simulink model "L1ZR5_Regelstrecke_inputgain_Modell_FRNEU"  (Simulink 7.8)
settings: Solver=ode45  StartTime=0.0  StopTime=10  FixedStep=6e-4
values from neighbouring files (symbols this model uses):
  Am = [0 1; -1/T^2 -2*xi/T]    [L1ZR5_Regelstrecke1_inputgain_Modell.m]    (also in Timedelaymargin.m = [0 1; -0.6400   -1.9200])
  b = [0;1]    [L1ZR5_Regelstrecke1_inputgain_Modell.m]    (also in Timedelaymargin.m)
  c = [1 0]    [L1ZR5_Regelstrecke1_inputgain_Modell.m]    (also in Timedelaymargin.m)
  epsilon = 1.3    [L1ZR5_Regelstrecke1_inputgain_Modell.m]
  epsilon_omega = 0.1    [L1ZR5_Regelstrecke1_inputgain_Modell.m]
  epsilon_sigma = 0.1    [L1ZR5_Regelstrecke1_inputgain_Modell.m]
  epsilon_theta = 0.1    [L1ZR5_Regelstrecke1_inputgain_Modell.m]
  Gamma = 100000000    [L1ZR5_Regelstrecke1_inputgain_Modell.m]
  ICy = 0    [L1ZR5_Regelstrecke1_inputgain_Modell.m]
  k = 1750    [L1ZR5_Regelstrecke1_inputgain_Modell.m]
  kg = -1/(c/Am*b)    [L1ZR5_Regelstrecke1_inputgain_Modell.m]
  KmY = 2.4    [L1ZR5_Regelstrecke1_inputgain_Modell.m]
  Kq = [(theta1_max+theta1_min)/2 (theta2_max+theta2_min)/2]    [L1ZR5_Regelstrecke1_inputgain_Modell.m]
  kvy = 0    [L1ZR5_Regelstrecke1_inputgain_Modell.m]
  m = 19    [L1ZR5_Regelstrecke1_inputgain_Modell.m]
  M = tf(ss(Am,bm,cm,0))    [L1ZR5_Regelstrecke1_inputgain_Modell.m]
  omega_max = omega0_max*1.2    (= 0.394105263158)    [L1ZR5_Regelstrecke1_inputgain_Modell.m]
  omega_min = omega0_min/1.2    (= 0.0311111111111)    [L1ZR5_Regelstrecke1_inputgain_Modell.m]
  omega_Pmax = (omega_max-omega_min)/2    (= 0.181497076023)    [L1ZR5_Regelstrecke1_inputgain_Modell.m]
  omega_Pr_Center = omega_Pmax + omega_min    (= 0.212608187135)    [L1ZR5_Regelstrecke1_inputgain_Modell.m]
  Pb = P*b    [L1ZR5_Regelstrecke1_inputgain_Modell.m]
  pD = p(2)-1.92    [L1ZR5_Regelstrecke1_inputgain_Modell.m]
  pI = p(4)    [L1ZR5_Regelstrecke1_inputgain_Modell.m]
  pK = p(3)-0.64    [L1ZR5_Regelstrecke1_inputgain_Modell.m]
  Ref_Amplitude = 0.3/Ref_Frequenz^2    (= 0.000303963550927)    [L1ZR5_Regelstrecke1_inputgain_Modell.m]
  Ref_Frequenz = 2*pi*5    (= 31.4159265359)    [L1ZR5_Regelstrecke1_inputgain_Modell.m]
  sigma_Pmax = Delta    (= 1000)    [L1ZR5_Regelstrecke1_inputgain_Modell.m]
  theta_Pmax = 2.56    [L1ZR5_Regelstrecke1_inputgain_Modell.m]
undefined symbols (not defined in the file or in its folder): d1, d2, delta, FpxLookUp1, FpxLookUp2, FpyLookUp1, FpyLookUp2, ICphi, ICvphi, ICvx, ICvy, ICx, J, KmX, kvphi, kvx, KX1, KX2, KY1, KY2, Ox1, Ox2, Oy1, Oy2, phx, phy, sigma, Tk, Vx1, Vx2, Vy1, Vy2, xLookUp1, xLookUp2, yLookUp1, yLookUp2
libraries: vrlib x6, simulink x3
settings Model: Creator=Markus  LastModifiedBy=Markus
settings SolverCC: ZeroCrossControl=EnableAll

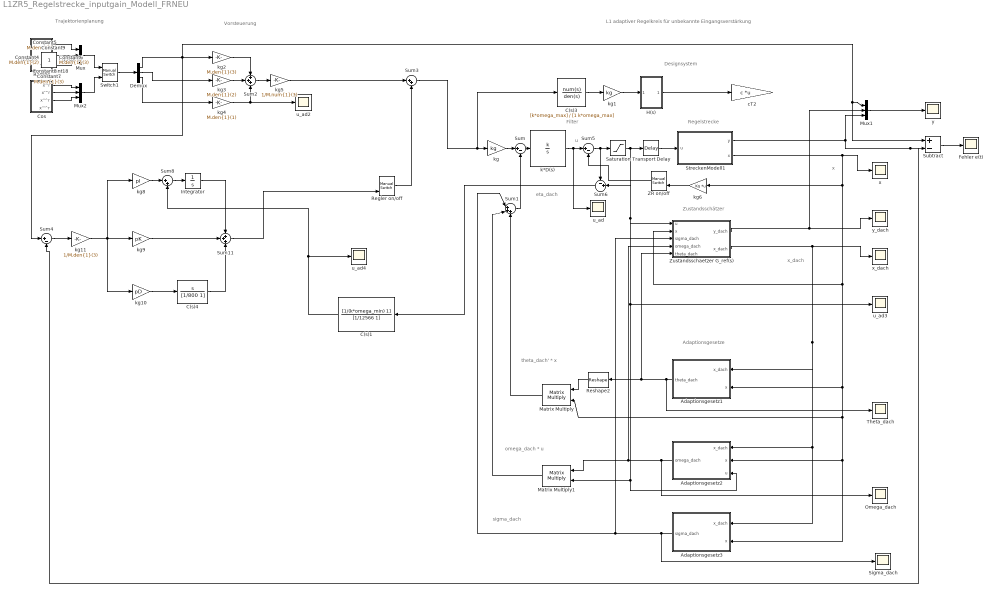
== system L1ZR5_Regelstrecke_inputgain_Modell_FRNEU ==
  note: Regelstrecke
  note: Zustandsschätzer
  note: Adaptionsgesetze
  note: L1 adaptiver Regelkreis für unbekannte Eingangsverstärkung
  note: x_dach
  note: x
  note: Filter
  note: u
  note: Designsystem
  note: theta_dach' * x
  note: omega_dach * u
  note: sigma_dach
  note: eta_dach
  note: Vorsteuerung
  note: Trajektorienplanung
  Adaptionsgesetz1 : Subsystem
  Adaptionsgesetz2 : Subsystem
  Adaptionsgesetz3 : Subsystem
  C(s)1 : TransferFcn  Numerator=[1/(k*omega_min) 1]  Denominator=[1/12566 1]
  C(s)3 : TransferFcn  Numerator=[k*omega_max]  Denominator=[1 k*omega_max]
  C(s)4 : TransferFcn  Numerator=[1 0]  Denominator=[1/800 1]
  Cos : Subsystem
  Demux : Demux  Outputs=3
  Fehler e(t) : Scope
      settings: TimeRange=4  YMin=-2.75e-005  YMax=2e-005  SaveName=simoutE
  H(s) : Subsystem
  Integrator : Integrator
  Matrix Multiply : Product  Multiplication=Matrix(*)
  Matrix Multiply1 : Product  Multiplication=Matrix(*)
  Mux : Mux  Inputs=3
  Mux1 : Mux  Inputs=3
  Mux2 : Mux  Inputs=3
  Omega_dach : Scope
      settings: TimeRange=0.01659605551497442  YMin=0.229945  YMax=0.254149  SaveName=simoutO
  Rampe : Subsystem
  Regler on/off : simulink/Signal Routing/Manual Switch  sw=0  action=0  varsize=off
  Reshape2 : Reshape  OutputDimensionality=Row vector (2-D)
  Saturation : Saturate  UpperLimit=20  LowerLimit=-20
  Sigma_dach : Scope
      settings: TimeRange=0.01659605551497442  YMin=0.18  YMax=0.25  SaveName=simoutS
  StreckenModell1 : Subsystem
  Subtract : Sum  Inputs=+-
  Sum : Sum  Inputs=|+-
  Sum1 : Sum  Inputs=|+++
  Sum11 : Sum  Inputs=+++
  Sum2 : Sum  Inputs=+++
  Sum3 : Sum  Inputs=|++
  Sum4 : Sum  Inputs=|+-
  Sum5 : Sum  Inputs=|+-
  Sum6 : Sum  Inputs=-+|
  Sum8 : Sum  Inputs=|++
  Switch1 : simulink/Signal Routing/Manual Switch  sw=1  action=0  varsize=off
  Theta_dach : Scope
      settings: TimeRange=0.01659605551497442  YMin=-0.05  YMax=0.275  SaveName=simoutT
  Transport Delay : TransportDelay  DelayTime=0.002
  ZR on/off : simulink/Signal Routing/Manual Switch  sw=1  action=0  varsize=off
  Zustandsschaetzer G_ref(s) : Subsystem
  cT2 : Gain  Gain=c  Multiplication=Matrix(K*u)
  k*D(s) : TransferFcn  Numerator=k  Denominator="[1  0]"
  kg : Gain  Gain=kg
  kg1 : Gain  Gain=kg
  kg10 : Gain  Gain=pD
  kg11 : Gain  Gain=1/M.den{1}(3)
  kg2 : Gain  Gain=M.den{1}(3)
  kg3 : Gain  Gain=M.den{1}(2)
  kg4 : Gain  Gain=M.den{1}(1)
  kg5 : Gain  Gain=1/M.num{1}(3)
  kg6 : Gain  Gain=Kq  Multiplication=Matrix(K*u)
  kg8 : Gain  Gain=pI
  kg9 : Gain  Gain=pK
  u_ad{,2..4} (4 alike) : Scope
      u_ad settings: TimeRange=4  YMin=-30  YMax=35  SaveName=simoutU
      u_ad2 settings: TimeRange=8  YMin=0.04404  YMax=0.04427  SaveName=simoutU2
      u_ad3 settings: TimeRange=4  YMin=-15  YMax=20  SaveName=simoutU3
      u_ad4 settings: TimeRange=20  YMin=-170  YMax=50  SaveName=simoutV2
  x : Scope
      settings: YMin=-0.0625  YMax=-0.005  SaveName=ScopeData3
  x_dach : Scope
      settings: YMin=-0.5  YMax=0.5  SaveName=ScopeData4
  y : Scope
      settings: TimeRange=4  YMin=-0.003  YMax=0.0015  SaveName=simout
  y_dach : Scope
      settings: YMin=0  YMax=35
  Constant{,1..3,8} (5 alike) : Constant  IOType=siggen  Value=k
  Constant18 : Constant  IOType=siggen
  Constant4 : Constant  IOType=siggen  Value=M.den{1}(2)
  Constant5 : Constant  IOType=siggen  Value=M.den{1}(2)
  Constant6 : Constant  IOType=siggen  Value=M.den{1}(3)
  Constant7 : Constant  IOType=siggen  Value=M.den{1}(3)
  Constant9 : Constant  IOType=siggen
  wires:
  kg/1 -> Sum/1
  Sum/1 -> k*D(s)/1
  Zustandsschaetzer G_ref(s)/1(y_dach) -> y_dach/1, Mux1/2
  StreckenModell1/1(y) -> Mux1/3, Subtract/2, Sum4/2
  StreckenModell1/2(x) -> x/1, Adaptionsgesetz1/2(x), Adaptionsgesetz2/2(x), Adaptionsgesetz3/2(x), Matrix Multiply/2, Zustandsschaetzer G_ref(s)/2(x), kg6/1
  Reshape2/1 -> Matrix Multiply/1
  Adaptionsgesetz1/1(theta_dach) -> Reshape2/1, Zustandsschaetzer G_ref(s)/5(theta_dach), Theta_dach/1
  Zustandsschaetzer G_ref(s)/2(x_dach) -> x_dach/1, Adaptionsgesetz1/1(x_dach), Adaptionsgesetz2/1(x_dach), Adaptionsgesetz3/1(x_dach)
  H(s)/1(Out1) -> cT2/1
  Mux1/1 -> y/1
  kg1/1 -> H(s)/1(In1)
  C(s)3/1 -> kg1/1
  Sum1/1 -> Sum/2
  Matrix Multiply/1 -> Sum1/3
  Adaptionsgesetz3/1(sigma_dach) -> Sum1/1, Zustandsschaetzer G_ref(s)/3(sigma_dach), Sigma_dach/1
  Adaptionsgesetz2/1(omega_dach) -> Zustandsschaetzer G_ref(s)/4(omega_dach), Matrix Multiply1/1, Omega_dach/1
  Matrix Multiply1/1 -> Sum1/2
  Demux/1 -> kg2/1, Mux1/1, Subtract/1, Sum4/1
  Demux/2 -> kg3/1
  Demux/3 -> kg4/1
  kg3/1 -> Sum2/2
  kg4/1 -> Sum2/3, u_ad2/1
  Sum2/1 -> kg5/1
  kg2/1 -> Sum2/1
  Rampe/1(y^r) -> Mux/1
  Rampe/2(y'^r) -> Mux/2
  Rampe/3(y''^r) -> Mux/3
  Mux/1 -> Switch1/1
  Switch1/1 -> Demux/1
  Mux2/1 -> Switch1/2
  Regler on/off/1 -> Sum3/2
  Sum6/1 -> C(s)1/1
  k*D(s)/1 -> Sum5/1, u_ad/1
  Saturation/1 -> Sum6/2, Transport Delay/1, Zustandsschaetzer G_ref(s)/1(u), u_ad3/1, Matrix Multiply1/2, Adaptionsgesetz2/3(u)
  Transport Delay/1 -> StreckenModell1/1(u)
  C(s)1/1 -> Sum8/2, u_ad4/1
  kg5/1 -> Sum3/1
  Cos/1(x^r) -> Mux2/1
  Cos/2(x'^r) -> Mux2/2
  Cos/3(x''^r) -> Mux2/3
  Sum3/1 -> kg/1, C(s)3/1
  Sum5/1 -> Sum6/1, Saturation/1
  Sum4/1 -> kg11/1
  Integrator/1 -> Sum11/1
  kg9/1 -> Sum11/2
  Sum11/1 -> Regler on/off/2
  kg8/1 -> Sum8/1
  Sum8/1 -> Integrator/1
  kg10/1 -> C(s)4/1
  C(s)4/1 -> Sum11/3
  kg11/1 -> kg8/1, kg9/1, kg10/1
  Subtract/1 -> Fehler e(t)/1
  kg6/1 -> ZR on/off/2
  ZR on/off/1 -> Sum5/2

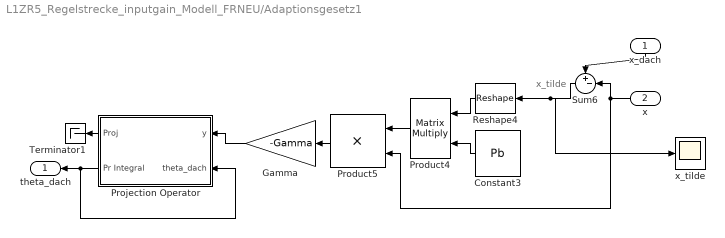
== system L1ZR5_Regelstrecke_inputgain_Modell_FRNEU/Adaptionsgesetz1 ==
  note: x_tilde
  x_dach : Inport
  x : Inport  Port=2
  Constant3 : Constant  Value=Pb
  Gamma : Gain  Gain=-Gamma
  Product4 : Product  Multiplication=Matrix(*)  RndMeth=Zero
  Product5 : Product  RndMeth=Zero
  Projection Operator : Subsystem  mask{EpsilonTheta=epsilon_theta, Prmax=theta_Pmax, Pr0=0}
      mask prompts: EpsilonTheta "Epsilon"; Prmax "Bound (radius of the ball)"; Pr0 "Initialization of integral"
      mask help:
      | Computes projection of the signal and safely integrate it.
      | Works both for scalar and vector signals.
      | It considers the parameter set as a ball at the origin with setted radius.
      mask init:
      | Thetamax = Prmax / sqrt(EpsilonTheta+1);
  Reshape4 : Reshape  OutputDimensionality=Row vector (2-D)
  Sum6 : Sum  Inputs=+-|
  Terminator1 : Terminator
  x_tilde : Scope
      settings: YMin=0  YMax=35  SaveName=ScopeData2
  theta_dach : Outport
  wires:
  Sum6/1 -> Reshape4/1, x_tilde/1
  Reshape4/1 -> Product4/1
  Constant3/1 -> Product4/2
  Product4/1 -> Product5/1
  Product5/1 -> Gamma/1
  Gamma/1 -> Projection Operator/1(y)
  Projection Operator/2(Pr Integral) -> theta_dach/1, Projection Operator/2(theta_dach)
  Projection Operator/1(Proj) -> Terminator1/1
  x_dach/1 -> Sum6/1
  x/1 -> Sum6/2, Product5/2

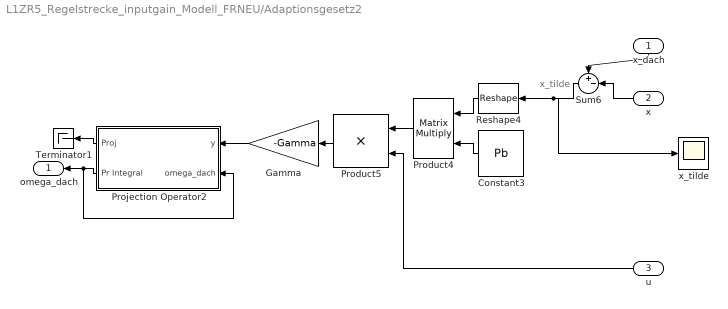
== system L1ZR5_Regelstrecke_inputgain_Modell_FRNEU/Adaptionsgesetz2 ==
  note: x_tilde
  x_dach : Inport
  x : Inport  Port=2
  u : Inport  Port=3
  Constant3 : Constant  Value=Pb
  Gamma : Gain  Gain=-Gamma
  Product4 : Product  Multiplication=Matrix(*)  RndMeth=Zero
  Product5 : Product  RndMeth=Zero
  Projection Operator2 : Subsystem  AncestorBlock=Projection/Projection Operator  mask{EpsilonTheta=epsilon_omega, Prmax=omega_Pmax, Prcenter=omega_Pr_Center, Pr0=omega_Pr_Center}
      mask prompts: EpsilonTheta "Epsilon"; Prmax "Bound (radius of the ball)"; Prcenter "Center of the Ball"; Pr0 "Initialization of integral"
      mask help:
      | Computes projection of the signal and safely integrate it.
      | Works both for scalar and vector signals.
      | It considers the parameter set as a ball at the specified location with
      | preset radius.
      mask init:
      | Thetamax = Prmax / sqrt(EpsilonTheta+1);
      | Intmax = Prmax+Prcenter;
      | Intmin = -Prmax+Prcenter;
  Reshape4 : Reshape  OutputDimensionality=Row vector (2-D)
  Sum6 : Sum  Inputs=+-|
  Terminator1 : Terminator
  x_tilde : Scope
      settings: YMin=0  YMax=35  SaveName=ScopeData2
  omega_dach : Outport
  wires:
  Sum6/1 -> Reshape4/1, x_tilde/1
  Reshape4/1 -> Product4/1
  Constant3/1 -> Product4/2
  Product4/1 -> Product5/1
  Product5/1 -> Gamma/1
  Gamma/1 -> Projection Operator2/1(y)
  Projection Operator2/2(Pr Integral) -> omega_dach/1, Projection Operator2/2(omega_dach)
  Projection Operator2/1(Proj) -> Terminator1/1
  x_dach/1 -> Sum6/1
  x/1 -> Sum6/2
  u/1 -> Product5/2

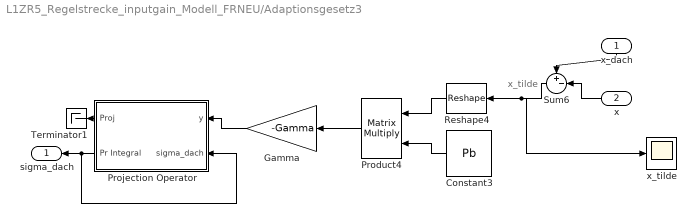
== system L1ZR5_Regelstrecke_inputgain_Modell_FRNEU/Adaptionsgesetz3 ==
  note: x_tilde
  x_dach : Inport
  x : Inport  Port=2
  Constant3 : Constant  Value=Pb
  Gamma : Gain  Gain=-Gamma
  Product4 : Product  Multiplication=Matrix(*)  RndMeth=Zero
  Projection Operator : Subsystem  mask{EpsilonTheta=epsilon_sigma, Prmax=sigma_Pmax, Pr0=0}
      mask prompts: EpsilonTheta "Epsilon"; Prmax "Bound (radius of the ball)"; Pr0 "Initialization of integral"
      mask help:
      | Computes projection of the signal and safely integrate it.
      | Works both for scalar and vector signals.
      | It considers the parameter set as a ball at the origin with setted radius.
      mask init:
      | Thetamax = Prmax / sqrt(EpsilonTheta+1);
  Reshape4 : Reshape  OutputDimensionality=Row vector (2-D)
  Sum6 : Sum  Inputs=+-|
  Terminator1 : Terminator
  x_tilde : Scope
      settings: YMin=0  YMax=35  SaveName=ScopeData2
  sigma_dach : Outport
  wires:
  Sum6/1 -> Reshape4/1, x_tilde/1
  Reshape4/1 -> Product4/1
  Constant3/1 -> Product4/2
  Gamma/1 -> Projection Operator/1(y)
  Projection Operator/2(Pr Integral) -> sigma_dach/1, Projection Operator/2(sigma_dach)
  Projection Operator/1(Proj) -> Terminator1/1
  x_dach/1 -> Sum6/1
  x/1 -> Sum6/2
  Product4/1 -> Gamma/1

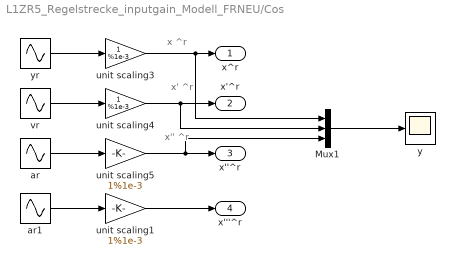
== system L1ZR5_Regelstrecke_inputgain_Modell_FRNEU/Cos ==
  note: x ^r
  note: x' ^r
  note: x'' ^r
  Mux1 : Mux  Inputs=3
  ar : Sin  Amplitude=-Ref_Amplitude*Ref_Frequenz^2  Frequency=Ref_Frequenz  Phase=pi/2  SampleTime=0
  ar1 : Sin  Amplitude=Ref_Amplitude*Ref_Frequenz^3  Frequency=Ref_Frequenz  SampleTime=0
  unit scaling1 : Gain  Gain=1%1e-3
  unit scaling3 : Gain  Gain=1 %1e-3
  unit scaling4 : Gain  Gain=1 %1e-3
  unit scaling5 : Gain  Gain=1%1e-3
  vr : Sin  Amplitude=-Ref_Amplitude*Ref_Frequenz  Frequency=Ref_Frequenz  SampleTime=0
  y : Scope
      settings: TimeRange=20  YMin=-0.3  YMax=0.8  SaveName=simout1
  yr : Sin  Amplitude=Ref_Amplitude  Frequency=Ref_Frequenz  Phase=pi/2  SampleTime=0
  x^r : Outport
  x'^r : Outport  Port=2
  x''^r : Outport  Port=3
  x'''^r : Outport  Port=4
  wires:
  ar/1 -> unit scaling5/1
  vr/1 -> unit scaling4/1
  yr/1 -> unit scaling3/1
  unit scaling3/1 -> x^r/1, Mux1/1
  unit scaling4/1 -> x'^r/1, Mux1/2
  unit scaling5/1 -> x''^r/1, Mux1/3
  Mux1/1 -> y/1
  ar1/1 -> unit scaling1/1
  unit scaling1/1 -> x'''^r/1

== system L1ZR5_Regelstrecke_inputgain_Modell_FRNEU/H(s) ==
  In1 : Inport
  Am2 : Gain  Gain=Am  Multiplication=Matrix(K*u)
  Integrator2 : Integrator
  Sum5 : Sum  Inputs=|++
  b2 : Gain  Gain=b  Multiplication=Matrix(K*u)
  Out1 : Outport
  wires:
  Integrator2/1 -> Am2/1, Out1/1
  Sum5/1 -> Integrator2/1
  b2/1 -> Sum5/1
  Am2/1 -> Sum5/2
  In1/1 -> b2/1

== system L1ZR5_Regelstrecke_inputgain_Modell_FRNEU/Rampe ==
  note: y ^r
  note: y' ^r
  note: y'' ^r
  Integrator1 : Integrator  InitialCondition=ICvy
  Integrator4 : Integrator  InitialCondition=ICy
  Mux1 : Mux  Inputs=3
  Scaling of a_max : Gain  Gain=300/500
  ays : FromWorkspace  VariableName=[t ays]  SampleTime=0
  unit scaling : Gain  Gain=1e-3
  y : Scope
      settings: TimeRange=20  YMin=-0.005  YMax=0.07  SaveName=simout2
  y^r : Outport
  y'^r : Outport  Port=2
  y''^r : Outport  Port=3
  wires:
  ays/1 -> Scaling of a_max/1
  Scaling of a_max/1 -> unit scaling/1
  Integrator1/1 -> Integrator4/1, y'^r/1, Mux1/2
  unit scaling/1 -> Integrator1/1, y''^r/1, Mux1/3
  Integrator4/1 -> y^r/1, Mux1/1
  Mux1/1 -> y/1

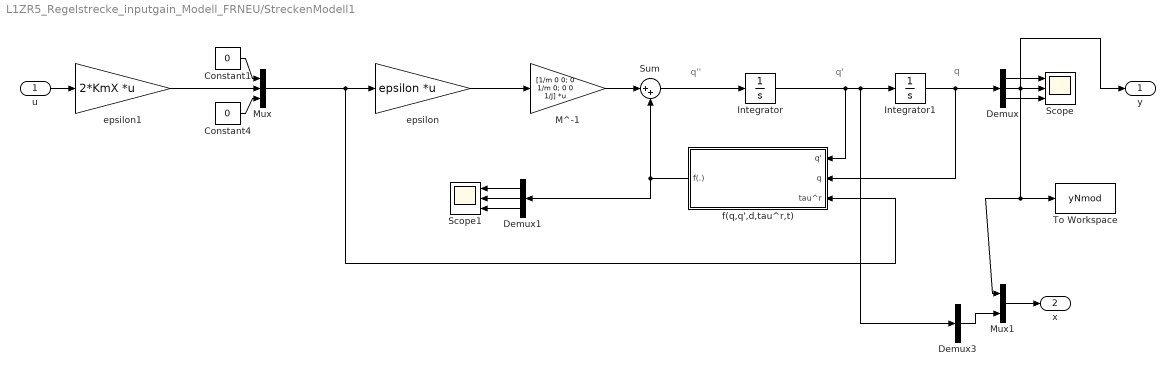
== system L1ZR5_Regelstrecke_inputgain_Modell_FRNEU/StreckenModell1 ==
  note: q
  note: q'
  note: q''
  u : Inport
  Constant1 : Constant  Value=0
  Constant4 : Constant  Value=0
  Demux : Demux  Outputs=3
  Demux1 : Demux  Outputs=3
  Demux3 : Demux  Outputs=3
  Integrator : Integrator  InitialCondition=[ICvx;ICvy;ICvphi]
  Integrator1 : Integrator  InitialCondition=[ICx;ICy;ICphi]
  M^-1 : Gain  Gain=[1/m 0 0; 0 1/m 0; 0 0 1/J]  Multiplication=Matrix(K*u)
  Mux : Mux  Inputs=3
  Mux1 : Mux  Inputs=2
  Scope : Scope  NumInputPorts=3
      settings: YMin=0.0014~0.0425~-1.73472e-018  YMax=0.0029~0.0625~0.08
  Scope1 : Scope  NumInputPorts=3
      settings: YMin=-1~1.1~-1  YMax=1~2.6~1  SaveName=ScopeData2
  Sum : Sum  Inputs=|++
  To Workspace : ToWorkspace  VariableName=yNmod  SampleTime=-1  SaveFormat=Structure With Time
  epsilon : Gain  Gain=epsilon  Multiplication=Matrix(K*u)
  epsilon1 : Gain  Gain=2*KmX  Multiplication=Matrix(K*u)
  f(q,q',d,tau^r,t) : Subsystem
  y : Outport
  x : Outport  Port=2
  wires:
  Demux3/2 -> Mux1/2
  Mux1/1 -> x/1
  Constant4/1 -> Mux/3
  Constant1/1 -> Mux/1
  Mux/1 -> f(q,q',d,tau^r,t)/3(tau^r), epsilon/1
  Demux1/3 -> Scope1/3
  Demux1/2 -> Scope1/2
  Demux1/1 -> Scope1/1
  f(q,q',d,tau^r,t)/1(f(.)) -> Demux1/1, Sum/2
  epsilon/1 -> M^-1/1
  Integrator1/1 -> f(q,q',d,tau^r,t)/2(q), Demux/1
  Sum/1 -> Integrator/1
  M^-1/1 -> Sum/1
  Integrator/1 -> Demux3/1, Integrator1/1, f(q,q',d,tau^r,t)/1(q')
  Demux/3 -> Scope/3
  Demux/2 -> Mux1/1, To Workspace/1, y/1, Scope/2
  Demux/1 -> Scope/1
  u/1 -> epsilon1/1
  epsilon1/1 -> Mux/2

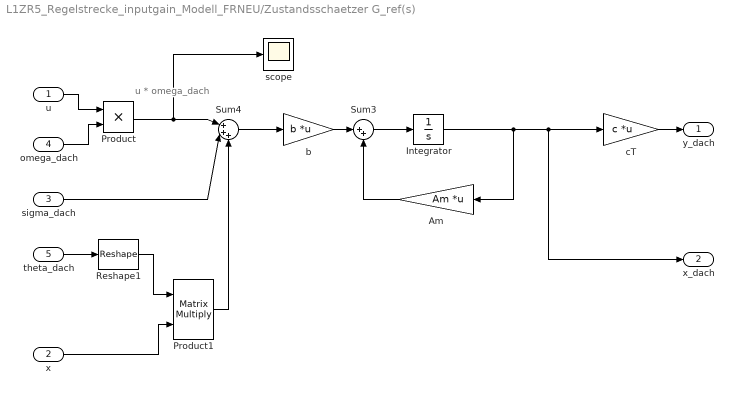
== system L1ZR5_Regelstrecke_inputgain_Modell_FRNEU/Zustandsschaetzer G_ref(s) ==
  note: u * omega_dach
  u : Inport
  x : Inport  Port=2
  sigma_dach : Inport  Port=3
  omega_dach : Inport  Port=4
  theta_dach : Inport  Port=5
  Am : Gain  Gain=Am  Multiplication=Matrix(K*u)
  Integrator : Integrator
  Product : Product  RndMeth=Zero
  Product1 : Product  Multiplication=Matrix(*)  RndMeth=Zero
  Reshape1 : Reshape  OutputDimensionality=Row vector (2-D)
  Sum3 : Sum  Inputs=|++
  Sum4 : Sum  Inputs=|+++
  b : Gain  Gain=b  Multiplication=Matrix(K*u)
  cT : Gain  Gain=c  Multiplication=Matrix(K*u)
  scope : Scope
      settings: TimeRange=15  YMin=-1  SaveName=ScopeData17
  y_dach : Outport
  x_dach : Outport  Port=2
  wires:
  Integrator/1 -> Am/1, cT/1, x_dach/1
  Sum3/1 -> Integrator/1
  b/1 -> Sum3/1
  Am/1 -> Sum3/2
  cT/1 -> y_dach/1
  Reshape1/1 -> Product1/1
  theta_dach/1 -> Reshape1/1
  omega_dach/1 -> Product/2
  u/1 -> Product/1
  Sum4/1 -> b/1
  Product1/1 -> Sum4/3
  Product/1 -> Sum4/1, scope/1
  sigma_dach/1 -> Sum4/2
  x/1 -> Product1/2

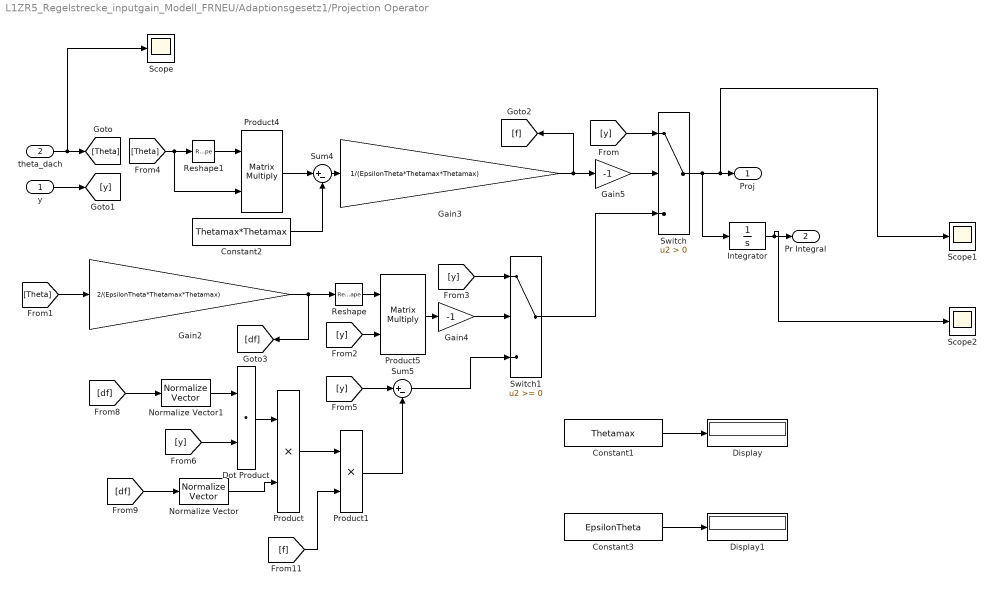
== system L1ZR5_Regelstrecke_inputgain_Modell_FRNEU/Adaptionsgesetz1/Projection Operator ==
  y : Inport
  theta_dach : Inport  Port=2
  Constant1 : Constant  Value=Thetamax  VectorParams1D=off
  Constant2 : Constant  Value=Thetamax*Thetamax
  Constant3 : Constant  Value=EpsilonTheta  VectorParams1D=off
  Display : Display
  Display1 : Display
  Dot Product : DotProduct  InputSameDT=on  OutDataTypeStr=Inherit: Inherit via internal rule
  Gain2 : Gain  Gain=2/(EpsilonTheta*Thetamax*Thetamax)
  Gain3 : Gain  Gain=1/(EpsilonTheta*Thetamax*Thetamax)
  Gain4 : Gain  Gain=-1
  Gain5 : Gain  Gain=-1
  Integrator : Integrator  InitialCondition=Pr0  LimitOutput=on  UpperSaturationLimit=Prmax  LowerSaturationLimit=-Prmax
  Normalize Vector : vrlib/Utilities/Normalize Vector  maxzero=0
  Normalize Vector1 : vrlib/Utilities/Normalize Vector  maxzero=0
  Product : Product  RndMeth=Zero
  Product1 : Product  RndMeth=Zero
  Product4 : Product  Multiplication=Matrix(*)  RndMeth=Zero
  Product5 : Product  Multiplication=Matrix(*)  RndMeth=Zero
  Reshape : Reshape  OutputDimensionality=Row vector (2-D)
  Reshape1 : Reshape  OutputDimensionality=Row vector (2-D)
  Scope : Scope
      settings: YMin=-6  YMax=9  SaveName=ScopeData8
  Scope1 : Scope
      settings: YMin=-150000  YMax=150000  SaveName=ScopeData9
  Scope2 : Scope
      settings: YMin=-6  YMax=9  SaveName=ScopeData10
  Sum4 : Sum  Inputs=|+-
  Sum5 : Sum  Inputs=|+-
  Switch : Switch  Criteria=u2 > Threshold
  Switch1 : Switch
  Proj : Outport
  Pr Integral : Outport  Port=2
  wires:
  Gain5/1 -> Switch/2
  Sum5/1 -> Switch1/3
  [y] -> Sum5/1
  theta_dach/1 -> [Theta], Scope/1
  y/1 -> [y]
  Switch/1 -> Integrator/1, Proj/1, Scope1/1
  Switch1/1 -> Switch/3
  [Theta] -> Gain2/1
  [y] -> Switch1/1
  Gain4/1 -> Switch1/2
  Product5/1 -> Gain4/1
  [y] -> Product5/2
  [y] -> Switch/1
  Gain3/1 -> [f], Gain5/1
  Sum4/1 -> Gain3/1
  Constant2/1 -> Sum4/2
  [Theta] -> Reshape1/1, Product4/2
  Gain2/1 -> Reshape/1, [df]
  Reshape/1 -> Product5/1
  Reshape1/1 -> Product4/1
  [df] -> Normalize Vector1/1
  [df] -> Normalize Vector/1
  Normalize Vector1/1 -> Dot Product/1
  [y] -> Dot Product/2
  Dot Product/1 -> Product/1
  Normalize Vector/1 -> Product/2
  Product/1 -> Product1/1
  [f] -> Product1/2
  Product1/1 -> Sum5/2
  Integrator/1 -> Pr Integral/1, Scope2/1
  Constant1/1 -> Display/1
  Constant3/1 -> Display1/1
  Product4/1 -> Sum4/1

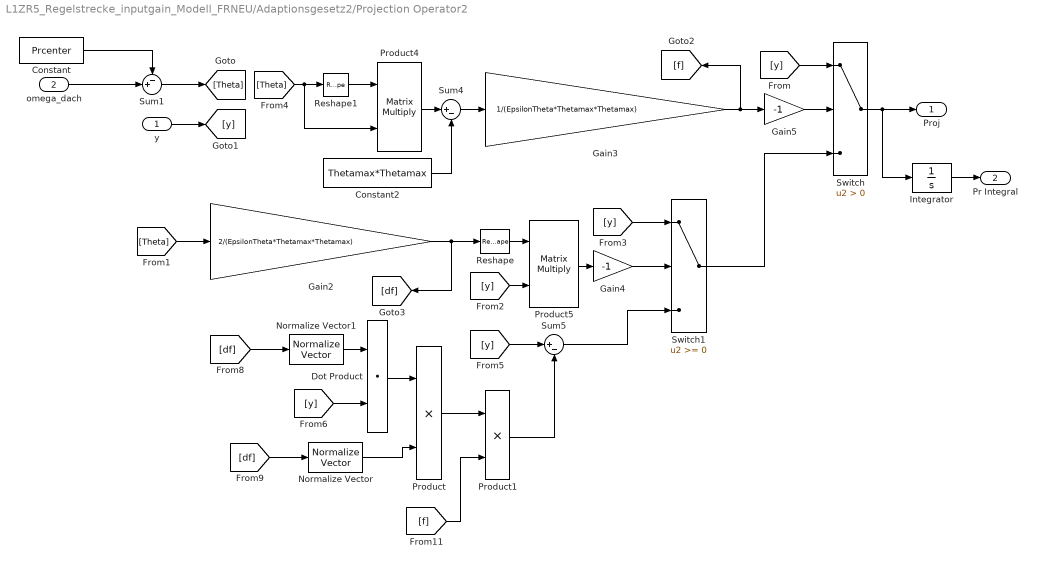
== system L1ZR5_Regelstrecke_inputgain_Modell_FRNEU/Adaptionsgesetz2/Projection Operator2 ==
  y : Inport
  omega_dach : Inport  Port=2
  Constant : Constant  Value=Prcenter
  Constant2 : Constant  Value=Thetamax*Thetamax
  Dot Product : DotProduct  InputSameDT=on  OutDataTypeStr=Inherit: Inherit via internal rule
  Gain2 : Gain  Gain=2/(EpsilonTheta*Thetamax*Thetamax)
  Gain3 : Gain  Gain=1/(EpsilonTheta*Thetamax*Thetamax)
  Gain4 : Gain  Gain=-1
  Gain5 : Gain  Gain=-1
  Integrator : Integrator  InitialCondition=Pr0  LimitOutput=on  UpperSaturationLimit=Intmax  LowerSaturationLimit=Intmin
  Normalize Vector : vrlib/Utilities/Normalize Vector  maxzero=0
  Normalize Vector1 : vrlib/Utilities/Normalize Vector  maxzero=0
  Product : Product  RndMeth=Zero
  Product1 : Product  RndMeth=Zero
  Product4 : Product  Multiplication=Matrix(*)  RndMeth=Zero
  Product5 : Product  Multiplication=Matrix(*)  RndMeth=Zero
  Reshape : Reshape  OutputDimensionality=Row vector (2-D)
  Reshape1 : Reshape  OutputDimensionality=Row vector (2-D)
  Sum1 : Sum  Inputs=-+|
  Sum4 : Sum  Inputs=|+-
  Sum5 : Sum  Inputs=|+-
  Switch : Switch  Criteria=u2 > Threshold
  Switch1 : Switch
  Proj : Outport
  Pr Integral : Outport  Port=2
  wires:
  Constant/1 -> Sum1/1
  Sum1/1 -> [Theta]
  omega_dach/1 -> Sum1/2
  Integrator/1 -> Pr Integral/1
  Product1/1 -> Sum5/2
  [f] -> Product1/2
  Product/1 -> Product1/1
  Normalize Vector/1 -> Product/2
  Dot Product/1 -> Product/1
  [y] -> Dot Product/2
  Normalize Vector1/1 -> Dot Product/1
  [df] -> Normalize Vector/1
  [df] -> Normalize Vector1/1
  Reshape1/1 -> Product4/1
  Reshape/1 -> Product5/1
  Gain2/1 -> [df], Reshape/1
  [Theta] -> Product4/2, Reshape1/1
  Product4/1 -> Sum4/1
  Constant2/1 -> Sum4/2
  Sum4/1 -> Gain3/1
  Gain3/1 -> Gain5/1, [f]
  [y] -> Switch/1
  [y] -> Product5/2
  Product5/1 -> Gain4/1
  Gain4/1 -> Switch1/2
  [y] -> Switch1/1
  [Theta] -> Gain2/1
  Switch1/1 -> Switch/3
  Switch/1 -> Integrator/1, Proj/1
  y/1 -> [y]
  [y] -> Sum5/1
  Sum5/1 -> Switch1/3
  Gain5/1 -> Switch/2

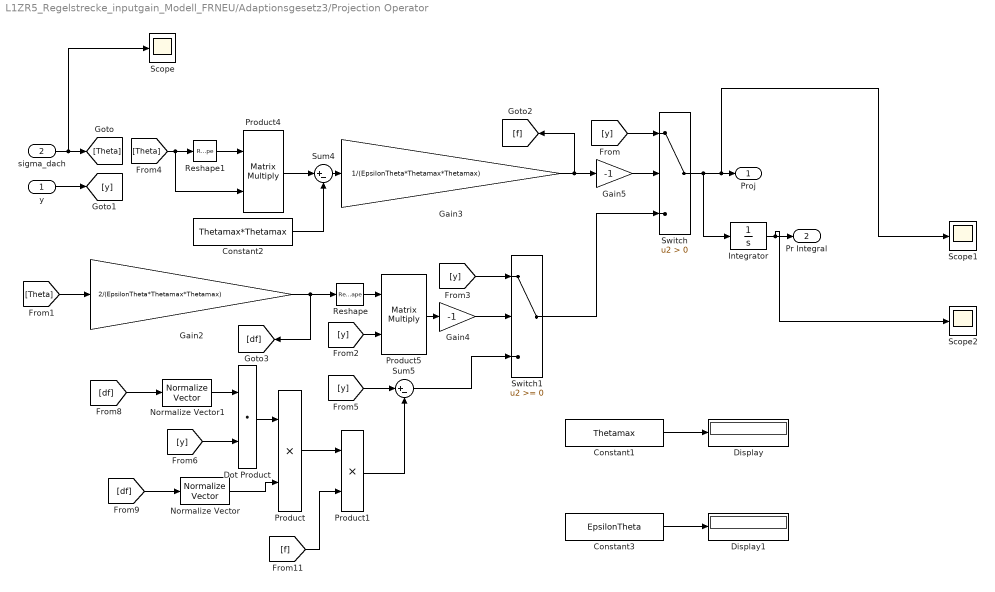
== system L1ZR5_Regelstrecke_inputgain_Modell_FRNEU/Adaptionsgesetz3/Projection Operator ==
  y : Inport
  sigma_dach : Inport  Port=2
  Constant1 : Constant  Value=Thetamax  VectorParams1D=off
  Constant2 : Constant  Value=Thetamax*Thetamax
  Constant3 : Constant  Value=EpsilonTheta  VectorParams1D=off
  Display : Display
  Display1 : Display
  Dot Product : DotProduct  InputSameDT=on  OutDataTypeStr=Inherit: Inherit via internal rule
  Gain2 : Gain  Gain=2/(EpsilonTheta*Thetamax*Thetamax)
  Gain3 : Gain  Gain=1/(EpsilonTheta*Thetamax*Thetamax)
  Gain4 : Gain  Gain=-1
  Gain5 : Gain  Gain=-1
  Integrator : Integrator  InitialCondition=Pr0  LimitOutput=on  UpperSaturationLimit=Prmax  LowerSaturationLimit=-Prmax
  Normalize Vector : vrlib/Utilities/Normalize Vector  maxzero=0
  Normalize Vector1 : vrlib/Utilities/Normalize Vector  maxzero=0
  Product : Product  RndMeth=Zero
  Product1 : Product  RndMeth=Zero
  Product4 : Product  Multiplication=Matrix(*)  RndMeth=Zero
  Product5 : Product  Multiplication=Matrix(*)  RndMeth=Zero
  Reshape : Reshape  OutputDimensionality=Row vector (2-D)
  Reshape1 : Reshape  OutputDimensionality=Row vector (2-D)
  Scope : Scope
      settings: YMin=-6  YMax=9  SaveName=ScopeData8
  Scope1 : Scope
      settings: YMin=-150000  YMax=150000  SaveName=ScopeData9
  Scope2 : Scope
      settings: YMin=-6  YMax=9  SaveName=ScopeData10
  Sum4 : Sum  Inputs=|+-
  Sum5 : Sum  Inputs=|+-
  Switch : Switch  Criteria=u2 > Threshold
  Switch1 : Switch
  Proj : Outport
  Pr Integral : Outport  Port=2
  wires:
  Gain5/1 -> Switch/2
  Sum5/1 -> Switch1/3
  [y] -> Sum5/1
  sigma_dach/1 -> [Theta], Scope/1
  y/1 -> [y]
  Switch/1 -> Integrator/1, Proj/1, Scope1/1
  Switch1/1 -> Switch/3
  [Theta] -> Gain2/1
  [y] -> Switch1/1
  Gain4/1 -> Switch1/2
  Product5/1 -> Gain4/1
  [y] -> Product5/2
  [y] -> Switch/1
  Gain3/1 -> [f], Gain5/1
  Sum4/1 -> Gain3/1
  Constant2/1 -> Sum4/2
  [Theta] -> Reshape1/1, Product4/2
  Gain2/1 -> Reshape/1, [df]
  Reshape/1 -> Product5/1
  Reshape1/1 -> Product4/1
  [df] -> Normalize Vector1/1
  [df] -> Normalize Vector/1
  Normalize Vector1/1 -> Dot Product/1
  [y] -> Dot Product/2
  Dot Product/1 -> Product/1
  Normalize Vector/1 -> Product/2
  Product/1 -> Product1/1
  [f] -> Product1/2
  Product1/1 -> Sum5/2
  Integrator/1 -> Pr Integral/1, Scope2/1
  Constant1/1 -> Display/1
  Constant3/1 -> Display1/1
  Product4/1 -> Sum4/1

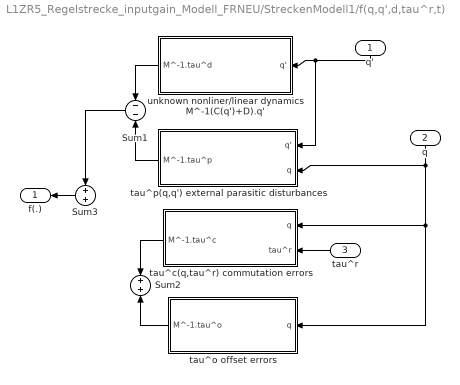
== system L1ZR5_Regelstrecke_inputgain_Modell_FRNEU/StreckenModell1/f(q,q',d,tau^r,t) ==
  q' : Inport
  q : Inport  Port=2
  tau^r : Inport  Port=3
  Sum1 : Sum  Inputs=--
  Sum2 : Sum
  Sum3 : Sum
  tau^c(q,tau^r) commutation errors : Subsystem
  tau^o offset errors : Subsystem
  tau^p(q,q') external parasitic disturbances : Subsystem
  unknown nonliner/linear dynamics M^-1(C(q')+D).q' : Subsystem
  f(.) : Outport
  wires:
  Sum3/1 -> f(.)/1
  tau^r/1 -> tau^c(q,tau^r) commutation errors/2(tau^r)
  q/1 -> tau^o offset errors/1(q), tau^c(q,tau^r) commutation errors/1(q), tau^p(q,q') external parasitic disturbances/2(q)
  q'/1 -> unknown nonliner/linear dynamics M^-1(C(q')+D).q'/1(q'), tau^p(q,q') external parasitic disturbances/1(q')
  unknown nonliner/linear dynamics M^-1(C(q')+D).q'/1(M^-1.tau^d) -> Sum1/1
  tau^c(q,tau^r) commutation errors/1(M^-1.tau^c) -> Sum2/1
  tau^o offset errors/1(M^-1.tau^o) -> Sum2/2
  Sum1/1 -> Sum3/1
  tau^p(q,q') external parasitic disturbances/1(M^-1.tau^p) -> Sum1/2

== system L1ZR5_Regelstrecke_inputgain_Modell_FRNEU/StreckenModell1/f(q,q',d,tau^r,t)/tau^c(q,tau^r) commutation errors ==
  q : Inport
  tau^r : Inport  Port=2
  Co(x,y) : MATLAB Function  TreatAsAtomicUnit=on
  Delta_B(x,y) : MATLAB Function  TreatAsAtomicUnit=on
  "M^-1  " : Gain  Gain=[1/m 0 0; 0 1/m 0; 0 0 1/J]  Multiplication=Matrix(K*u)
  Matrix Multiply : Product  Multiplication=Matrix(*)
  Matrix Multiply1 : Product  Multiplication=Matrix(*)
  epsilon : Gain  Gain=epsilon  Multiplication=Matrix(K*u)
  M^-1.tau^c : Outport
  wires:
  "M^-1  "/1 -> epsilon/1
  epsilon/1 -> M^-1.tau^c/1
  tau^r/1 -> Matrix Multiply1/2
  q/1 -> Co(x,y)/1(q), Delta_B(x,y)/1(q)
  Matrix Multiply1/1 -> "M^-1  "/1
  Matrix Multiply/1 -> Matrix Multiply1/1
  Co(x,y)/1(Co) -> Matrix Multiply/2
  Delta_B(x,y)/1(Delta_B) -> Matrix Multiply/1

== system L1ZR5_Regelstrecke_inputgain_Modell_FRNEU/StreckenModell1/f(q,q',d,tau^r,t)/tau^o offset errors ==
  q : Inport
  Delta_B(x,y) : MATLAB Function  TreatAsAtomicUnit=on
  "M^-1  " : Gain  Gain=[1/m 0 0; 0 1/m 0; 0 0 1/J]  Multiplication=Matrix(K*u)
  Matrix Multiply1 : Product  Multiplication=Matrix(*)
  sigma : Constant  Value=sigma
  M^-1.tau^o : Outport
  wires:
  sigma/1 -> Matrix Multiply1/2
  Matrix Multiply1/1 -> "M^-1  "/1
  "M^-1  "/1 -> M^-1.tau^o/1
  q/1 -> Delta_B(x,y)/1(q)
  Delta_B(x,y)/1(Bp) -> Matrix Multiply1/1

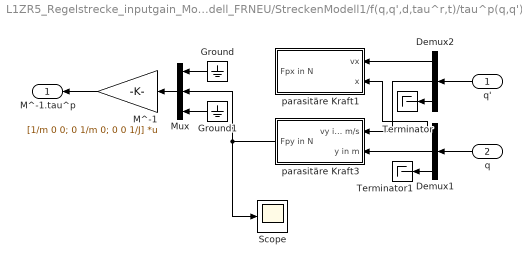
== system L1ZR5_Regelstrecke_inputgain_Modell_FRNEU/StreckenModell1/f(q,q',d,tau^r,t)/tau^p(q,q') external parasitic disturbances ==
  q' : Inport
  q : Inport  Port=2
  Demux1 : Demux  Outputs=3
  Demux2 : Demux  Outputs=3
  Ground : Ground
  Ground1 : Ground
  "M^-1  " : Gain  Gain=[1/m 0 0; 0 1/m 0; 0 0 1/J]  Multiplication=Matrix(K*u)
  Mux : Mux  Inputs=3
  Scope : Scope
      settings: YMin=-4.06576e-020  YMax=0.0007  SaveName=ScopeData19
  Terminator : Terminator
  Terminator1 : Terminator
  parasitäre Kraft1 : Subsystem
  parasitäre Kraft3 : Subsystem
  M^-1.tau^p : Outport
  wires:
  Ground1/1 -> Mux/3
  "M^-1  "/1 -> M^-1.tau^p/1
  Mux/1 -> "M^-1  "/1
  q/1 -> Demux1/1
  q'/1 -> Demux2/1
  parasitäre Kraft3/1(Fpy in N) -> Scope/1, Mux/2
  Demux2/2 -> parasitäre Kraft3/1(vy in m/s)
  Demux1/3 -> Terminator1/1
  Demux2/3 -> Terminator/1
  Demux2/1 -> parasitäre Kraft1/1(vx)
  Demux1/2 -> parasitäre Kraft3/2(y in m)
  Demux1/1 -> parasitäre Kraft1/2(x)
  Ground/1 -> Mux/1

== system L1ZR5_Regelstrecke_inputgain_Modell_FRNEU/StreckenModell1/f(q,q',d,tau^r,t)/unknown nonliner/linear dynamics M^-1(C(q')+D).q' ==
  q' : Inport
  C(q').q' : Subsystem
  "M^-1 " : Gain  Gain=[1/m 0 0; 0 1/m 0; 0 0 1/J]  Multiplication=Matrix(K*u)
  M^-1.D : Gain  Gain=[kvx/m 0 0; 0 kvy/m 0; 0 0 kvphi/J]  Multiplication=Matrix(K*u)
  Sum1 : Sum
  M^-1.tau^d : Outport
  wires:
  M^-1.D/1 -> Sum1/1
  Sum1/1 -> M^-1.tau^d/1
  "M^-1 "/1 -> Sum1/2
  q'/1 -> C(q').q'/1(q'), M^-1.D/1
  C(q').q'/1(C(q').q') -> "M^-1 "/1

== system L1ZR5_Regelstrecke_inputgain_Modell_FRNEU/StreckenModell1/f(q,q',d,tau^r,t)/tau^p(q,q') external parasitic disturbances/parasitäre Kraft1 ==
  note: Modellansatz für das Störkraftmodell in x-Richtung:
      |
      | F_{px} ( x, v_x )=1/2 [ tanh(  \delta  v_x ) + 1 ] F_{p}^{  +}(x)  -  1/2 [ tanh( \delta  v_x )  - 1 ]  F_{p}^{  -}(x)
      |
      | mit
      |
      | x    ... x-Position
      | v_x  ... x-Geschwindigkeit
      | \delta   ... Steigung der tanh-Funktion
      |
      | F_{p}^{  + }(x)          ... positionsabhängige Störkraft für Geschwindigkeiten v_x   >  0  (aus Look-Up-Table \rightarrow Stellsignalversuche )
      | F_{p}^{  - }(x)           ... positionsabhängige Störkraft für Geschwindigkeiten v_x   <  0  (aus Look-Up-Table \rightarrow Stellsignalversuche )
      | F_{px} ( x, v_x ) ...positions- und richtungsabhängige Störkraft
  note: Störkraftmodell für die x-Richtung
  vx : Inport
  x : Inport  Port=2
  Fcn : Fcn  Expr=(tanh(delta*u)+1)/2
  Fcn1 : Fcn  Expr=-(tanh(delta*u)-1)/2
  Product : Product  RndMeth=Zero
  Product1 : Product  RndMeth=Zero
  Sum : Sum
  parasitäre Kräfte in x-Richtung v < 0 : Lookup_n-D  NumberOfTableDimensions=1  BreakpointsForDimension1=fliplr(xLookUp2')*1e-3+Vx2  Table=fliplr(FpxLookUp2')*KX2+Ox2  InterpMethod=Cubic spline  RndMeth=Simplest  InputSameDT=on
  parasitäre Kräfte in x-Richtung v > 0 : Lookup_n-D  NumberOfTableDimensions=1  BreakpointsForDimension1=xLookUp1*1e-3+Vx1  Table=FpxLookUp1*KX1+Ox1  InterpMethod=Cubic spline  RndMeth=Simplest  InputSameDT=on
  Fpx in N : Outport
  wires:
  vx/1 -> Fcn1/1, Fcn/1
  Sum/1 -> Fpx in N/1
  Product/1 -> Sum/2
  Product1/1 -> Sum/1
  Fcn/1 -> Product1/2
  parasitäre Kräfte in x-Richtung v > 0/1 -> Product1/1
  Fcn1/1 -> Product/1
  parasitäre Kräfte in x-Richtung v < 0/1 -> Product/2
  x/1 -> parasitäre Kräfte in x-Richtung v < 0/1, parasitäre Kräfte in x-Richtung v > 0/1

== system L1ZR5_Regelstrecke_inputgain_Modell_FRNEU/StreckenModell1/f(q,q',d,tau^r,t)/tau^p(q,q') external parasitic disturbances/parasitäre Kraft3 ==
  note: Störkraftmodell für die y-Richtung
  note: Modellansatz für das Störkraftmodell in y-Richtung:
      |
      | F_{py} ( y, v_y )=1/2 [ tanh(  \delta  v_y ) + 1 ] F_{p}^{  +}(y)  -  1/2 [ tanh( \delta  v_y )  - 1 ]  F_{p}^{  -}(y)
      |
      | mit
      |
      | y    ... y-Position
      | v_y  ... y-Geschwindigkeit
      | \delta   ... Steigung der tanh-Funktion
      |
      | F_{p}^{  + }(y)          ... positionsabhängige Störkraft für Geschwindigkeiten v_y   >  0  (aus Look-Up-Table \rightarrow Stellsignalversuche )
      | F_{p}^{  - }(y)           ... positionsabhängige Störkraft für Geschwindigkeiten v_y   <  0  (aus Look-Up-Table \rightarrow Stellsignalversuche )
      | F_{py} ( y, v_y ) ...positions- und richtungsabhängige Störkraft
  vy in m/s : Inport
  y in m : Inport  Port=2
  Fcn : Fcn  Expr=(tanh(delta*u)+1)/2
  Fcn1 : Fcn  Expr=-(tanh(delta*u)-1)/2
  Product : Product  RndMeth=Zero
  Product1 : Product  RndMeth=Zero
  Sum : Sum
  parasitäre Kräfte in y-Richtung v < 0 : Lookup_n-D  NumberOfTableDimensions=1  BreakpointsForDimension1=fliplr(yLookUp2')*1e-3+Vy2  Table=fliplr(FpyLookUp2')*KY2+Oy2  InterpMethod=Cubic spline  RndMeth=Simplest  InputSameDT=on
  parasitäre Kräfte in y-Richtung v > 0 : Lookup_n-D  NumberOfTableDimensions=1  BreakpointsForDimension1=yLookUp1*1e-3+Vy1  Table=FpyLookUp1*KY1+Oy1  InterpMethod=Cubic spline  RndMeth=Simplest  InputSameDT=on
  Fpy in N : Outport
  wires:
  parasitäre Kräfte in y-Richtung v < 0/1 -> Product/2
  parasitäre Kräfte in y-Richtung v > 0/1 -> Product1/1
  Product/1 -> Sum/2
  Product1/1 -> Sum/1
  Fcn/1 -> Product1/2
  Fcn1/1 -> Product/1
  Sum/1 -> Fpy in N/1
  vy in m/s/1 -> Fcn/1, Fcn1/1
  y in m/1 -> parasitäre Kräfte in y-Richtung v > 0/1, parasitäre Kräfte in y-Richtung v < 0/1

== system L1ZR5_Regelstrecke_inputgain_Modell_FRNEU/StreckenModell1/f(q,q',d,tau^r,t)/unknown nonliner/linear dynamics M^-1(C(q')+D).q'/C(q').q' ==
  note: \phi'
  note: y'
  note: x'
  q' : Inport
  Demux : Demux  Outputs=3
  Gain : Gain  Gain=[0 -(1-m) 0; (1-m) 0 0; 0 0 0]
  Matrix Multiply : Product  Multiplication=Matrix(*)
  Terminator : Terminator
  Terminator1 : Terminator
  C(q').q' : Outport
  wires:
  Demux/3 -> Gain/1
  Matrix Multiply/1 -> C(q').q'/1
  Gain/1 -> Matrix Multiply/1
  Demux/2 -> Terminator1/1
  Demux/1 -> Terminator/1
  q'/1 -> Matrix Multiply/2, Demux/1

== matlab function StreckenModell1/f(q,q',d,tau^r,t)/tau^c(q,tau^r) commutation errors/Co(x,y) ==
  data: q input double; Co output double; Tk parameter double; KmX parameter double; KmY parameter double; phx parameter double; phy parameter double; d1 parameter double; d2 parameter double
function Co = compute_Co(q,Tk,KmX,KmY,phx,phy,d1,d2)
%#codegen
x=q(1);
y=q(2);

% Flussdichte entlang der x- und y-Richtungen
B1x=sin(2*pi/Tk*x+phx+pi/2); %+
B2x=cos(2*pi/Tk*x+phx-pi/2); %-
B1y=sin(2*pi/Tk*y+phy);
B2y=cos(2*pi/Tk*y+phy);


Co =[B1x/(2*KmX)    0         d1*KmX*B1x/(2*(d1^2*KmX^2+d2^2*KmY^2));
     B2x/(2*KmX)    0         d1*KmX*B2x/(2*(d1^2*KmX^2+d2^2*KmY^2));
     B1x/(2*KmX)    0        -d1*KmX*B1x/(2*(d1^2*KmX^2+d2^2*KmY^2));
     B2x/(2*KmX)    0        -d1*KmX*B2x/(2*(d1^2*KmX^2+d2^2*KmY^2));
        0        B1y/(2*KmY) -d2*KmY*B1y/(2*(d1^2*KmX^2+d2^2*KmY^2));
        0        B2y/(2*KmY) -d2*KmY*B2y/(2*(d1^2*KmX^2+d2^2*KmY^2));
        0        B1y/(2*KmY)  d2*KmY*B1y/(2*(d1^2*KmX^2+d2^2*KmY^2));
        0        B2y/(2*KmY)  d2*KmY*B2y/(2*(d1^2*KmX^2+d2^2*KmY^2))];

== matlab function StreckenModell1/f(q,q',d,tau^r,t)/tau^c(q,tau^r) commutation errors/Delta_B(x,y) ==
  data: q input double; Delta_B output double; Tk parameter double; KmX parameter double; KmY parameter double; phx parameter double; phy parameter double; d1 parameter double; d2 parameter double
function Delta_B = compute_Delta_B(q,Tk,KmX,KmY,phx,phy,d1,d2)
%#codegen
x=q(1);
y=q(2);

% Flussdichte entlang der x- und y-Richtungen
B1x=KmX*sin(2*pi/Tk*x+phx+pi/2); %+
B2x=KmX*cos(2*pi/Tk*x+phx-pi/2); %-
B1y=KmY*sin(2*pi/Tk*y+phy);
B2y=KmY*cos(2*pi/Tk*y+phy);

% nominelles Feld
B =[   B1x    B2x     B1x     B2x      0       0      0      0;
        0      0       0       0      B1y     B2y    B1y    B2y;
     d1*B1x d1*B2x -d1*B1x -d1*B2x -d2*B1y -d2*B2y d2*B1y d2*B2y];

 
% Fehlerhaftes Magnetfeld
maxBp=0.4704;
B1xp=0.4851*tanh(0.1877*sinh(3.104*B1x))/maxBp; 
B2xp=0.4851*tanh(0.1877*sinh(3.104*B2x))/maxBp; 
B1yp=0.4851*tanh(0.1877*sinh(3.104*B1y))/maxBp; 
B2yp=0.4851*tanh(0.1877*sinh(3.104*B2y))/maxBp; 

Bp =[   B1xp    B2xp    B1xp     B2xp      0       0       0       0;
         0       0       0        0       B1yp    B2yp    B1yp    B2yp;
     d1*B1xp d1*B2xp -d1*B1xp -d1*B2xp -d2*B1yp -d2*B2yp d2*B1yp d2*B2yp];
 
Delta_B=Bp-B;

== matlab function StreckenModell1/f(q,q',d,tau^r,t)/tau^o offset errors/Delta_B(x,y) ==
  data: q input double; Bp output double; Tk parameter double; KmX parameter double; KmY parameter double; phx parameter double; phy parameter double; d1 parameter double; d2 parameter double
function Bp = compute_Bp(q,Tk,KmX,KmY,phx,phy,d1,d2)
%#codegen
x=q(1);
y=q(2);

% Flussdichte entlang der x- und y-Richtungen
B1x=KmX*sin(2*pi/Tk*x+phx+pi/2); %+
B2x=KmX*cos(2*pi/Tk*x+phx-pi/2); %-
B1y=KmY*sin(2*pi/Tk*y+phy);
B2y=KmY*cos(2*pi/Tk*y+phy);
 
% Fehlerhaftes Magnetfeld
maxBp=0.4704;
B1xp=0.4851*tanh(0.1877*sinh(3.104*B1x))/maxBp; 
B2xp=0.4851*tanh(0.1877*sinh(3.104*B2x))/maxBp; 
B1yp=0.4851*tanh(0.1877*sinh(3.104*B1y))/maxBp; 
B2yp=0.4851*tanh(0.1877*sinh(3.104*B2y))/maxBp; 

Bp =[   B1xp    B2xp    B1xp     B2xp      0       0       0       0;
         0       0       0        0       B1yp    B2yp    B1yp    B2yp;
     d1*B1xp d1*B2xp -d1*B1xp -d1*B2xp -d2*B1yp -d2*B2yp d2*B1yp d2*B2yp];
